simulink model "Proyecto"  (R2022a)
settings: Solver=VariableStepAuto  StartTime=0.0  StopTime=10000000  RelTol=1e-3  EnableMultiTasking=on
undefined symbols (not defined in the file or in its folder): dvbs2ldpc
libraries: commblkcod2 x6, commchan3 x4, commdigbbndpm3 x4, commsink2 x4, commdigbbndam3 x4
settings Model: Creator=The MathWorks, Inc.  LastModifiedBy=danie
settings SolverCC: AlgebraicLoopSolver=TrustRegion
settings DataIOCC: LimitDataPoints=on  SaveFormat=Array  ReturnWorkspaceOutputs=off  SignalLoggingName=sigsOut
settings OptimizationCC: ExpressionDepthLimit=2147483647  InitFltsAndDblsToZero=on  LifeSpan=inf
settings DebuggingCC: SaveWithParameterizedLinksMsg=none  UnderspecifiedInitializationDetection=Classic  MergeDetectMultiDrivingBlocksExec=none  SignalResolutionControl=TryResolveAllWithWarning  MultiTaskDSMMsg=warning  MultiTaskCondExecSysMsg=none  FcnCallInpInsideContextMsg=warning  UnconnectedInputMsg=warning  UnconnectedOutputMsg=warning  UnconnectedLineMsg=warning  StateNameClashWarn=warning  SFUnexpectedBacktrackingDiag=warning  SFNoUnconditionalDefaultTransitionDiag=warning  SFExecutionAtInitializationDiag=none  SFMachineParentedDataDiag=warning  ArithmeticOperatorsInVariantConditions=warning
settings HardwareCC: ProdBitPerPointer=32  ProdBitPerSizeT=32  ProdBitPerPtrDiffT=32  ProdLargestAtomicFloat=None  ProdIntDivRoundTo=Undefined  ProdEndianess=Unspecified  ProdWordSize=32  ProdHWDeviceType=32-bit Generic  TargetUnknown=on
settings ModelReferenceCC: PropagateSignalLabelsOutOfModel=off
settings SFSimCC: SimUseLocalCustomCode=off  CustomCodeUndefinedFunction=UseInterfaceOnly
settings RTWCC: RTWUseLocalCustomCode=off  DLArmComputeVersion=19.05
settings CodeAppCC: StateflowObjectComments=on
settings GRTTargetCC: TargetFcnLib=ansi_tfl_tmw.mat  TargetLangStandard=C89/C90 (ANSI)  CombineOutputUpdateFcns=off  GRTInterface=on
settings ConfigComp: CovMetricSettings=dw  CovSaveCumulativeToWorkspaceVar=on  CovSaveSingleToWorkspaceVar=on  CovExternalEMLEnable=off

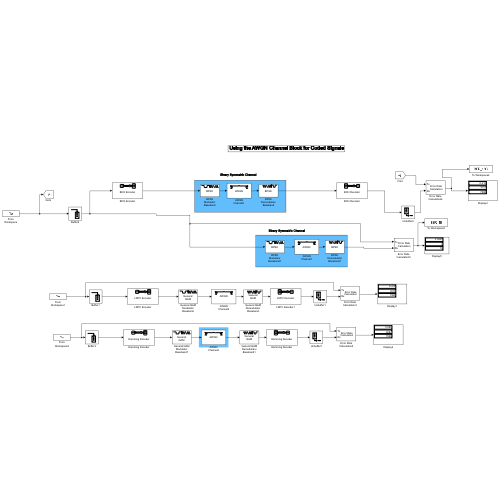
[thumbnail: Simulink's stored preview of the top-level diagram]
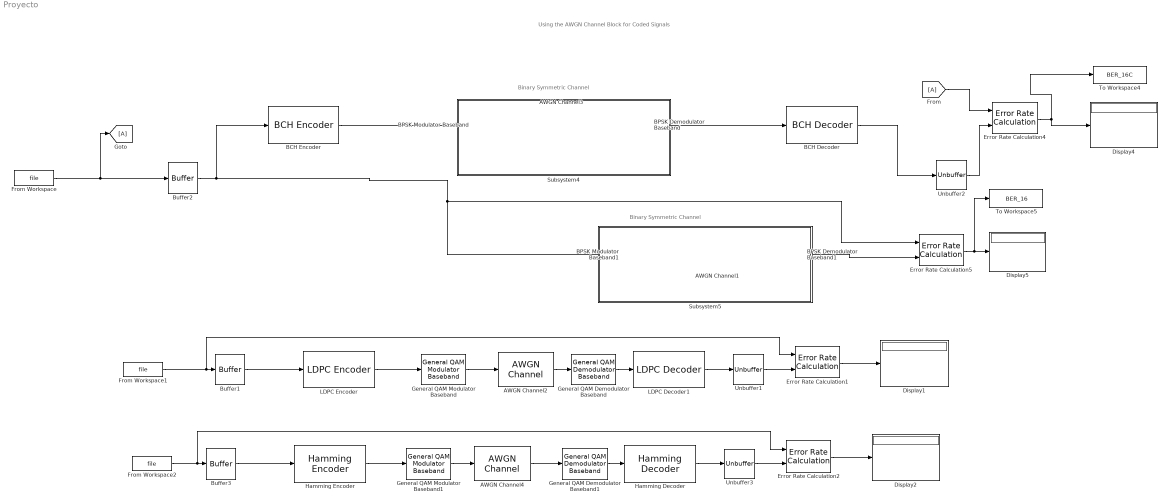
== system Proyecto ==
  note: Using the AWGN Channel Block for Coded Signals
  note: Binary Symmetric Channel
  note: Binary Symmetric Channel
  AWGN Channel1 : commchan3/AWGN Channel  InputProcessing=Columns as channels (frame based)  seed=67  noiseMode="Signal to noise ratio  (Eb/No)"  EbNodB=3  EsNodB=10  SNRdB=10  bitsPerSym=1  Ps=1  Tsym=1  variance=1
  AWGN Channel2 : commchan3/AWGN Channel  InputProcessing=Columns as channels (frame based)  seed=67  noiseMode="Signal to noise ratio  (Eb/No)"  EbNodB=3  EsNodB=10  SNRdB=10  bitsPerSym=1  Ps=2  Tsym=1  variance=1
  AWGN Channel3 : commchan3/AWGN Channel  InputProcessing=Columns as channels (frame based)  seed=67  noiseMode="Signal to noise ratio  (Eb/No)"  EbNodB=3  EsNodB=10  SNRdB=10  bitsPerSym=1  Ps=1  Tsym=1  variance=1
  AWGN Channel4 : commchan3/AWGN Channel  InputProcessing=Columns as channels (frame based)  seed=67  noiseMode="Signal to noise ratio  (Eb/No)"  EbNodB=3  EsNodB=10  SNRdB=10  bitsPerSym=1  Ps=1  Tsym=1  variance=1
  BCH Decoder : commblkcod2/BCH Decoder  n=31  k=16  specShortening=off  shortenedK=5  specGenPoly=off  genPoly='X^10 + X^8 + X^5 + X^4 + X^2 + X + 1'  specPrimPoly=off  prPoly='X^4 + X + 1'  specDisableGenCheck=off  specPuncture=off  punctVec=[ones(8,1); zeros(2,1)]  specErasurePort=off  showNumErr=off
      settings: SourceProductBaseCode=CM
  BCH Encoder : commblkcod2/BCH Encoder  n=31  k=16  specShortening=off  shortenedK=5  specGenPoly=off  genPoly='X^10 + X^8 + X^5 + X^4 + X^2 + X + 1'  specPrimPoly=off  prPoly='X^4 + X + 1'  specDisableGenCheck=off  specPuncture=off  punctVec=[ones(8,1); zeros(2,1)]
      settings: SourceProductBaseCode=CM
  BPSK Demodulator Baseband : commdigbbndpm3/BPSK Demodulator Baseband  DecType=Hard decision  VarSource=Dialog  Variance=1  Ph=0  outDtype=Inherit via internal rule  derotateFactorWordLen=16  derotateFactorDataTypeStr=Inherit: Same word length as input  derotateFactorLastDataTypeStr=Inherit: Same word length as input
  BPSK Demodulator Baseband1 : commdigbbndpm3/BPSK Demodulator Baseband  DecType=Hard decision  VarSource=Dialog  Variance=1  Ph=0  outDtype=Inherit via internal rule  derotateFactorWordLen=16  derotateFactorDataTypeStr=Inherit: Same word length as input  derotateFactorLastDataTypeStr=Inherit: Same word length as input
  BPSK Modulator Baseband : commdigbbndpm3/BPSK Modulator Baseband  Ph=0  outDtype=double  outWordLen=16  outUDDataType=sfix(16)  outFracLenMode=Best precision  outFracLen=15  outDataTypeStr=double  outLastDataTypeStr=double
  BPSK Modulator Baseband1 : commdigbbndpm3/BPSK Modulator Baseband  Ph=0  outDtype=double  outWordLen=16  outUDDataType=sfix(16)  outFracLenMode=Best precision  outFracLen=15  outDataTypeStr=double  outLastDataTypeStr=double
  Buffer1 : Buffer  N=32400  OutputFrames=off
  Buffer2 : Buffer  N=16  OutputFrames=off
  Buffer3 : Buffer  N=11  OutputFrames=off
  Display{1..2,4..5} (4 alike) : Display
  Error Rate Calculation{1..2,4..5} (4 alike) : commsink2/Error Rate Calculation  N=0  st_delay=0  cp_mode=Entire frame  subframe=[]  PMode=Port  WsName=ErrorVec  RsMode2=off  stop=on  numErr=200  maxBits=1e6
  From : From
  From Workspace : FromWorkspace  VariableName=file  SampleTime=1
  From Workspace1 : FromWorkspace  VariableName=file  SampleTime=1/1e6
  From Workspace2 : FromWorkspace  VariableName=file  SampleTime=1/1e6
  General QAM Demodulator Baseband : commdigbbndam3/General QAM Demodulator Baseband  SigCon=[exp(2*pi*1i*[0:63]/64)]  OutType=Integer  DecType=Hard decision  VarSource=Dialog  Variance=1  outDtypeBit=Inherit via internal rule  outDtype=Inherit via internal rule  roundingMode=Floor  overflowMode=Wrap  OvFlMode=off  OvFlModeLastStrValue=off  sigConstWordLen=16  sigConstDataTypeStr=Inherit: Same word length as input  sigConstLastDataTypeStr=Inherit: Same word length as input  accum1WordLen=32  accum1FracLen=30  prodInWordLen=32  prodInFracLen=30  prodInDataTypeStr=Inherit: Same as accumulator 1  prodInLastDataTypeStr=Inherit: Same as accumulator 1  prodOutWordLen=32  prodOutFracLen=30  accum2WordLen=32  accum2FracLen=30  accum3WordLen=32  accum3FracLen=30  nsiWordLen=32  nsiFracLen=30  nsiDataTypeStr=Inherit: Same as accumulator 3  nsiLastDataTypeStr=Inherit: Same as accumulator 3  invn0WordLen=16  invn0FracLen=8  invn0DataTypeStr=Inherit: Same word length as input  invn0LastDataTypeStr=Inherit: Same word length as input  outputWordLen=32  outputFracLen=30
      settings: SourceProductBaseCode=CM
  General QAM Demodulator Baseband1 : commdigbbndam3/General QAM Demodulator Baseband  SigCon=[exp(2*pi*1i*[0:63]/64)]  OutType=Integer  DecType=Hard decision  VarSource=Dialog  Variance=1  outDtypeBit=Inherit via internal rule  outDtype=Inherit via internal rule  roundingMode=Floor  overflowMode=Wrap  OvFlMode=off  OvFlModeLastStrValue=off  sigConstWordLen=16  sigConstDataTypeStr=Inherit: Same word length as input  sigConstLastDataTypeStr=Inherit: Same word length as input  accum1WordLen=32  accum1FracLen=30  prodInWordLen=32  prodInFracLen=30  prodInDataTypeStr=Inherit: Same as accumulator 1  prodInLastDataTypeStr=Inherit: Same as accumulator 1  prodOutWordLen=32  prodOutFracLen=30  accum2WordLen=32  accum2FracLen=30  accum3WordLen=32  accum3FracLen=30  nsiWordLen=32  nsiFracLen=30  nsiDataTypeStr=Inherit: Same as accumulator 3  nsiLastDataTypeStr=Inherit: Same as accumulator 3  invn0WordLen=16  invn0FracLen=8  invn0DataTypeStr=Inherit: Same word length as input  invn0LastDataTypeStr=Inherit: Same word length as input  outputWordLen=32  outputFracLen=30
      settings: SourceProductBaseCode=CM
  General QAM Modulator Baseband : commdigbbndam3/General QAM Modulator Baseband  SigCon=[exp(2*pi*1i*[0:63]/64)]  outDtype=double  outWordLen=16  outUDDataType=sfix(16)  outFracLenMode=Best precision  outFracLen=15  outDataTypeStr=double  outLastDataTypeStr=double
      settings: SourceProductBaseCode=CM
  General QAM Modulator Baseband1 : commdigbbndam3/General QAM Modulator Baseband  SigCon=[exp(2*pi*1i*[0:63]/64)]  outDtype=double  outWordLen=16  outUDDataType=sfix(16)  outFracLenMode=Best precision  outFracLen=15  outDataTypeStr=double  outLastDataTypeStr=double
      settings: SourceProductBaseCode=CM
  Goto : Goto
  Hamming Decoder : commblkcod2/Hamming Decoder  n=15  k=11
      settings: SourceProductBaseCode=CM
  Hamming Encoder : commblkcod2/Hamming Encoder  n=15  k=11
      settings: SourceProductBaseCode=CM
  LDPC Decoder1 : commblkcod2/LDPC Decoder  ParityCheckMat=dvbs2ldpc(1/2)  OutputFmt=Information part  DecisionType=Hard decision  OutputDataType=double  NumIter=50  DoParityCheck=off  OutputNumIter=off  OutputFinalChecks=off
      settings: SourceProductBaseCode=CM
  LDPC Encoder : commblkcod2/LDPC Encoder  ParityCheckMat=dvbs2ldpc(1/2)
      settings: SourceProductBaseCode=CM
  Subsystem4 : Subsystem
      mask Display: disp('')
  Subsystem5 : Subsystem
      mask Display: disp('')
  To Workspace4 : ToWorkspace  VariableName=BER_16C  SaveFormat=Timeseries  SampleTime=-1
  To Workspace5 : ToWorkspace  VariableName=BER_16  SaveFormat=Timeseries  SampleTime=-1
  Unbuffer1 : Unbuffer
  Unbuffer2 : Unbuffer
  Unbuffer3 : Unbuffer
  wires:
  BPSK Demodulator Baseband1/1 -> Error Rate Calculation5/2
  Error Rate Calculation4/1 -> To Workspace4/1, Display4/1
  Error Rate Calculation5/1 -> To Workspace5/1, Display5/1
  Buffer2/1 -> BCH Encoder/1, BPSK Modulator Baseband1/1, Error Rate Calculation5/1
  BPSK Modulator Baseband/1 -> AWGN Channel3/1
  AWGN Channel3/1 -> BPSK Demodulator Baseband/1
  BCH Decoder/1 -> Unbuffer2/1
  Unbuffer2/1 -> Error Rate Calculation4/2
  AWGN Channel1/1 -> BPSK Demodulator Baseband1/1
  BPSK Modulator Baseband1/1 -> AWGN Channel1/1
  From Workspace/1 -> Goto/1, Buffer2/1
  BPSK Demodulator Baseband/1 -> BCH Decoder/1
  From/1 -> Error Rate Calculation4/1
  BCH Encoder/1 -> BPSK Modulator Baseband/1
  Buffer1/1 -> LDPC Encoder/1
  LDPC Encoder/1 -> General QAM Modulator Baseband/1
  General QAM Modulator Baseband/1 -> AWGN Channel2/1
  AWGN Channel2/1 -> General QAM Demodulator Baseband/1
  General QAM Demodulator Baseband/1 -> LDPC Decoder1/1
  LDPC Decoder1/1 -> Unbuffer1/1
  Unbuffer1/1 -> Error Rate Calculation1/2
  Error Rate Calculation1/1 -> Display1/1
  From Workspace2/1 -> Error Rate Calculation2/1, Buffer3/1
  General QAM Modulator Baseband1/1 -> AWGN Channel4/1
  Unbuffer3/1 -> Error Rate Calculation2/2
  General QAM Demodulator Baseband1/1 -> Hamming Decoder/1
  Hamming Decoder/1 -> Unbuffer3/1
  Error Rate Calculation2/1 -> Display2/1
  AWGN Channel4/1 -> General QAM Demodulator Baseband1/1
  Buffer3/1 -> Hamming Encoder/1
  Hamming Encoder/1 -> General QAM Modulator Baseband1/1
  From Workspace1/1 -> Error Rate Calculation1/1, Buffer1/1

== system Proyecto/Subsystem4 ==

== system Proyecto/Subsystem5 ==
